simulink model "simulink_model"  (R2022b)
settings: Solver=VariableStepAuto  StartTime=0.0  StopTime=3  RelTol=1e-3
values from neighbouring files (symbols this model uses):
  K1 = wn^2    [M2.m]
  K2 = 2*K1 - 2*zeta*wn    [M2.m]
  wn = pi/(tp*sqrt(1-zeta^2))    [M2.m]
  zeta = sqrt((a-1)/(a-2))    [M2.m]
settings Model: Creator=ThinkPad  LastModifiedBy=ThinkPad

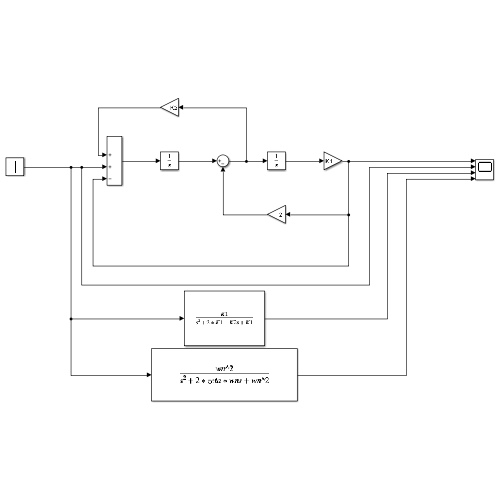
[thumbnail: Simulink's stored preview of the top-level diagram]
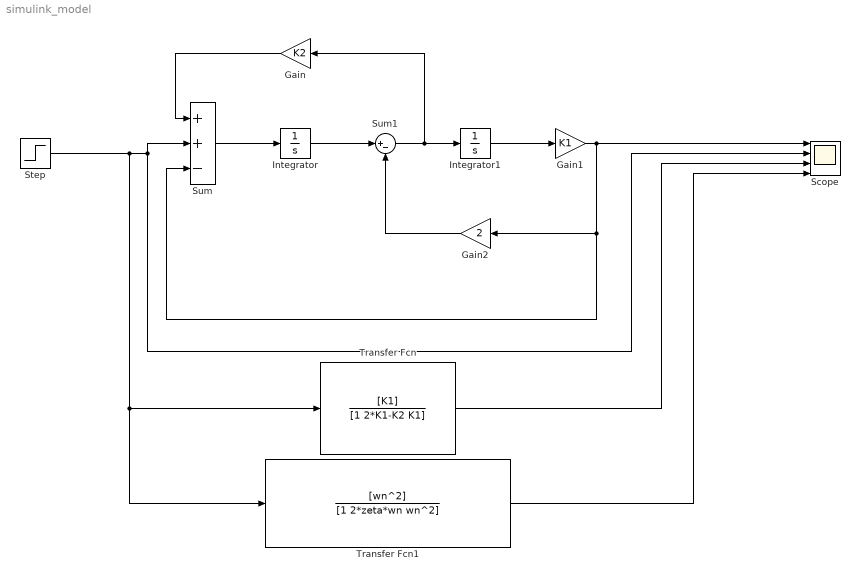
== system simulink_model ==
  Gain : Gain  Gain=K2
  Gain1 : Gain  Gain=K1
  Gain2 : Gain  Gain=2
  Integrator : Integrator
  Integrator1 : Integrator
  Scope : Scope  NumInputPorts=4
  Step : Step  Time=0  SampleTime=0
  Sum : Sum  Inputs=|++-
  Sum1 : Sum  Inputs=|+-
  Transfer Fcn : TransferFcn  Numerator=[K1]  Denominator=[1 2*K1-K2 K1]
  Transfer Fcn1 : TransferFcn  Numerator=[wn^2]  Denominator=[1 2*zeta*wn wn^2]
  wires:
  Step/1 -> Transfer Fcn/1, Transfer Fcn1/1, Scope/2, Sum/2
  Sum/1 -> Integrator/1
  Integrator/1 -> Sum1/1
  Gain/1 -> Sum/1
  Sum1/1 -> Gain/1, Integrator1/1
  Integrator1/1 -> Gain1/1
  Gain1/1 -> Sum/3, Gain2/1, Scope/1
  Gain2/1 -> Sum1/2
  Transfer Fcn/1 -> Scope/3
  Transfer Fcn1/1 -> Scope/4
